simulink model "lab10_observe_controller"  (Simulink 9.3)
settings: Solver=ode45  StartTime=0.0  StopTime=20.0  MaxStep=0.2  RelTol=1e-3  EnableMultiTasking=on
settings Model: Creator=qm-zhu  LastModifiedBy=qm-zhu
settings DataIOCC: LimitDataPoints=on
settings OptimizationCC: ExpressionDepthLimit=2147483647  InitFltsAndDblsToZero=on
settings DebuggingCC: SaveWithParameterizedLinksMsg=none  SignalResolutionControl=TryResolveAllWithWarning  SolverPrmCheckMsg=warning  MultiTaskDSMMsg=warning  MultiTaskCondExecSysMsg=none  StateNameClashWarn=warning
settings SFSimCC: SimUseLocalCustomCode=on
settings RTWCC: RTWUseLocalCustomCode=on
settings GRTTargetCC: TargetFcnLib=ansi_tfl_tmw.mat
settings ConfigComp: CovExternalEMLEnable=on

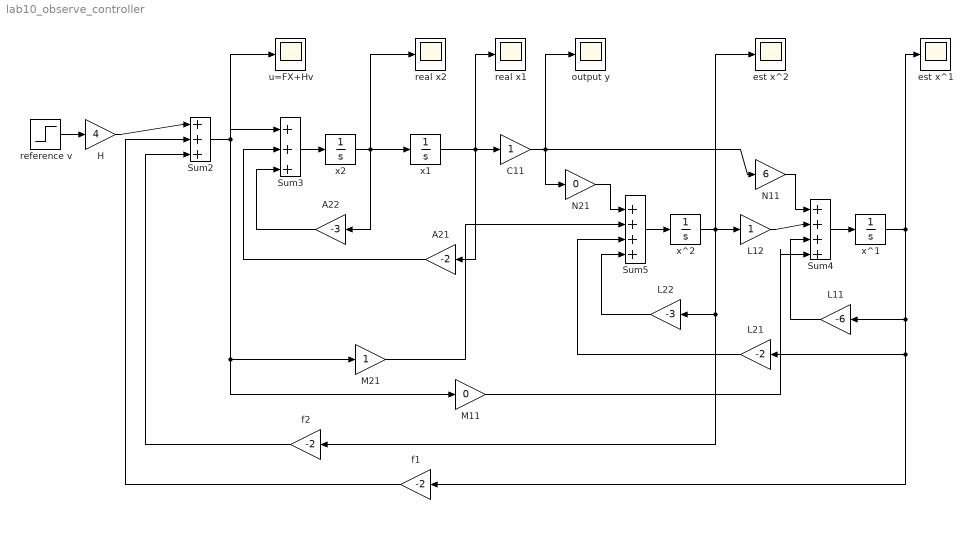
== system lab10_observe_controller ==
  A21 : Gain  Gain=-2
  A22 : Gain  Gain=-3
  C11 : Gain
  H : Gain  Gain=4
  L11 : Gain  Gain=-6
  L12 : Gain
  L21 : Gain  Gain=-2
  L22 : Gain  Gain=-3
  M11 : Gain  Gain=0
  M21 : Gain
  N11 : Gain  Gain=6
  N21 : Gain  Gain=0
  Sum2 : Sum  Inputs=|+++
  Sum3 : Sum  Inputs=|+++
  Sum4 : Sum  Inputs=|++++
  Sum5 : Sum  Inputs=|++++
  est x^1 : Scope
  est x^2 : Scope
  f1 : Gain  Gain=-2
  f2 : Gain  Gain=-2
  output y : Scope
  real x1 : Scope
  real x2 : Scope
  reference v : Step  SampleTime=0
  u=FX+Hv : Scope
  x1 : Integrator
  x2 : Integrator
  x^1 : Integrator
  x^2 : Integrator
  wires:
  reference v/1 -> H/1
  C11/1 -> output y/1, N21/1, N11/1
  f2/1 -> Sum2/3
  f1/1 -> Sum2/2
  H/1 -> Sum2/1
  Sum2/1 -> u=FX+Hv/1, M21/1, M11/1, Sum3/1
  Sum4/1 -> x^1/1
  x^1/1 -> L11/1, L21/1, f1/1, est x^1/1
  N11/1 -> Sum4/1
  L12/1 -> Sum4/2
  L11/1 -> Sum4/3
  Sum5/1 -> x^2/1
  x^2/1 -> L12/1, L22/1, f2/1, est x^2/1
  L21/1 -> Sum5/3
  M21/1 -> Sum5/2
  L22/1 -> Sum5/4
  N21/1 -> Sum5/1
  M11/1 -> Sum4/4
  x2/1 -> x1/1, A22/1, real x2/1
  x1/1 -> C11/1, A21/1, real x1/1
  A22/1 -> Sum3/3
  A21/1 -> Sum3/2
  Sum3/1 -> x2/1
